simulink model "Tut19_MergeBlock"  (R2021a)
settings: Solver=VariableStepAuto  StartTime=0.0  StopTime=10.0  RelTol=1e-3
settings Model: Creator=cheta  LastModifiedBy=cheta

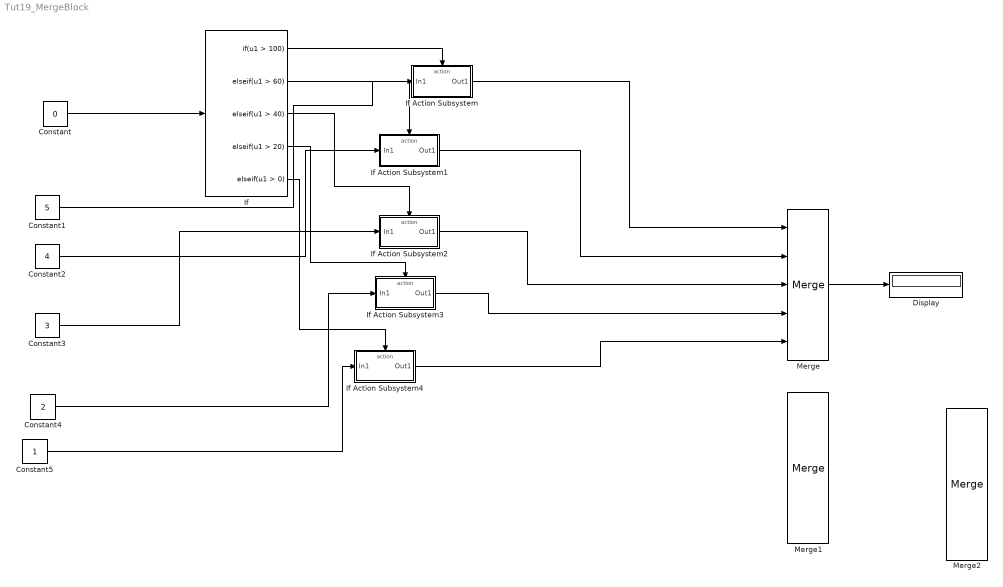
== system Tut19_MergeBlock ==
  Constant : Constant  Value=0
  Constant1 : Constant  Value=5
  Constant2 : Constant  Value=4
  Constant3 : Constant  Value=3
  Constant4 : Constant  Value=2
  Constant5 : Constant
  Display : Display
  If : If  IfExpression=u1 > 100  ElseIfExpressions=u1 > 60, u1 > 40, u1 > 20, u1 > 0  ShowElse=off
  If Action Subsystem : Subsystem  TreatAsAtomicUnit=on
  If Action Subsystem1 : Subsystem  TreatAsAtomicUnit=on
  If Action Subsystem2 : Subsystem  TreatAsAtomicUnit=on
  If Action Subsystem3 : Subsystem  TreatAsAtomicUnit=on
  If Action Subsystem4 : Subsystem  TreatAsAtomicUnit=on
  Merge : Merge  Inputs=5
  Merge1 : Merge  Inputs=5
  Merge2 : Merge  Inputs=5
  wires:
  Constant/1 -> If/1
  If/1 -> If Action Subsystem/Action
  If/2 -> If Action Subsystem1/Action
  If/3 -> If Action Subsystem2/Action
  If/4 -> If Action Subsystem3/Action
  If/5 -> If Action Subsystem4/Action
  Constant1/1 -> If Action Subsystem/1(In1)
  Constant2/1 -> If Action Subsystem1/1(In1)
  Constant3/1 -> If Action Subsystem2/1(In1)
  Constant4/1 -> If Action Subsystem3/1(In1)
  Constant5/1 -> If Action Subsystem4/1(In1)
  Merge/1 -> Display/1
  If Action Subsystem/1(Out1) -> Merge/1
  If Action Subsystem1/1(Out1) -> Merge/2
  If Action Subsystem2/1(Out1) -> Merge/3
  If Action Subsystem3/1(Out1) -> Merge/4
  If Action Subsystem4/1(Out1) -> Merge/5

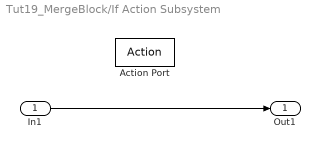
== system Tut19_MergeBlock/If Action Subsystem ==
  In1 : Inport
  Action Port : ActionPort  ActionPortLabel=if(u1 > 100)
  Out1 : Outport
  wires:
  In1/1 -> Out1/1

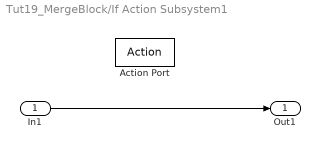
== system Tut19_MergeBlock/If Action Subsystem1 ==
  In1 : Inport
  Action Port : ActionPort  ActionPortLabel=elseif(u1 > 60)
  Out1 : Outport
  wires:
  In1/1 -> Out1/1

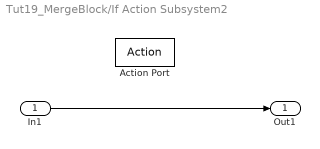
== system Tut19_MergeBlock/If Action Subsystem2 ==
  In1 : Inport
  Action Port : ActionPort  ActionPortLabel=elseif( u1 > 40)
  Out1 : Outport
  wires:
  In1/1 -> Out1/1

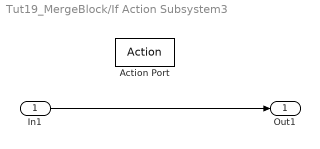
== system Tut19_MergeBlock/If Action Subsystem3 ==
  In1 : Inport
  Action Port : ActionPort  ActionPortLabel=elseif( u1 > 20)
  Out1 : Outport
  wires:
  In1/1 -> Out1/1

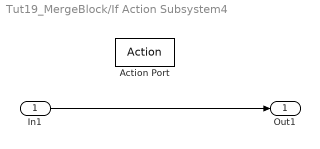
== system Tut19_MergeBlock/If Action Subsystem4 ==
  In1 : Inport
  Action Port : ActionPort  ActionPortLabel=elseif( u1 > 0)
  Out1 : Outport
  wires:
  In1/1 -> Out1/1
